simulink model "msfuntmpl_anfis1"  (Simulink 7.9)
settings: Solver=ode45  StartTime=0.0  StopTime=10.0  RelTol=1e-3
values from neighbouring files (symbols this model uses):
  a = dec2bin(J1(i,j))    [and2image.m]    (also in gncheck.m = imread('onion.png'); hist_eq.m = (l-1)/(m*n); histeq.m = (l-1)/(m*n))
  b = dec2bin(J2(i,j))    [and2image.m]    (also in boudary_extraction.m = stlm; fdatest.m = firpm(N, Fo, Ao, W, {dens}))
settings Model: Creator=NIRMAL  LastModifiedBy=NIRMAL
settings GRTTargetCC: CombineOutputUpdateFcns=off  GRTInterface=on

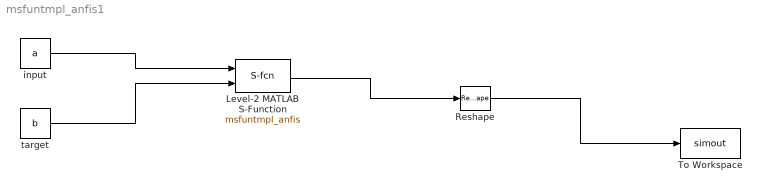
== system msfuntmpl_anfis1 ==
  Level-2 MATLAB S-Function : M-S-Function  FunctionName=msfuntmpl_anfis
  Reshape : Reshape  OutputDimensionality=Customize  OutputDimensions=[12,1]
  To Workspace : ToWorkspace  VariableName=simout  SampleTime=1
      settings: MaxDataPoints=1
  input : Constant  Value=a  VectorParams1D=off  OutDataTypeStr=double  SampleTime=1  LockScale=on
  target : Constant  Value=b  VectorParams1D=off  OutDataTypeStr=double  SampleTime=1  LockScale=on
  wires:
  input/1 -> Level-2 MATLAB S-Function/1
  target/1 -> Level-2 MATLAB S-Function/2
  Level-2 MATLAB S-Function/1 -> Reshape/1
  Reshape/1 -> To Workspace/1
